simulink model "clv3d"  (Simulink 8.4)
settings: Solver=ode45  SolverMode=SingleTasking  StartTime=0.0  StopTime=30  RelTol=1e-3  AbsTol=1e-6
settings Model: Creator=The MathWorks Inc.  LastModifiedBy=gcampa  ExtModeTrigMode=oneshot  ExtModeArmWhenConnect=off
settings DataIOCC: ExternalInput=[]  InitialState=[]  LimitDataPoints=off  SaveOutput=off  SaveTime=off
settings OptimizationCC: BlockReduction=off  BooleanDataType=off  ExpressionDepthLimit=128  InitFltsAndDblsToZero=on
settings DebuggingCC: SaveWithParameterizedLinksMsg=none  SignalResolutionControl=TryResolveAllWithWarning  SolverPrmCheckMsg=none  MultiTaskDSMMsg=warning  MultiTaskCondExecSysMsg=none  IntegerOverflowMsg=none  FcnCallInpInsideContextMsg=EnableAllAsError  FrameProcessingCompatibilityMsg=error  StateNameClashWarn=none
settings HardwareCC: TargetUnknown=on
settings GRTTargetCC: TargetFcnLib=ansi_tfl_tmw.mat
settings ConfigComp: CovMetricSettings=dw  CovHtmlReporting=on  CovSaveCumulativeToWorkspaceVar=on  CovSaveSingleToWorkspaceVar=on  CovModelRefEnable=Off  CovExternalEMLEnable=off  CovSFcnEnable=off

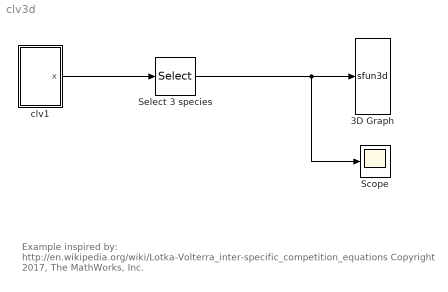
== system clv3d ==
  note: Example inspired by:
      | http://en.wikipedia.org/wiki/Lotka-Volterra_inter-specific_competition_equations
      | Copyright 2017, The MathWorks, Inc.
  3D Graph : S-Function  LoadFcn=if exist('sfun3d','file'), sfun3d([],[],[],'LoadBlock'); end  FunctionName=sfun3d  Parameters=ax,T,np,cp,gd,ls,mk,mx,hd,tb  EnableBusSupport=off  mask(3D Graph){np=1, ax=[0 1 0 1 0 0.5], mx=1e4, T=0.01, cp=[3 2 1], gd=on, hd=on, tb=on, ls=-, mk=none}
      mask prompts: np "Number of moving points (lines)"; ax "Range: [xmin xmax  ymin ymax zmin zmax]"; mx "Max number of points in each line"; T "Sampling Time"; cp "Camera position (use [0 0 1] for 2D XY view)"; gd "Grid (on|off)"; hd "HeadMarkers (on|off)"; tb "Toolbar (on|off)"; ls "LineStyle"; mk "LineMarker"
      mask help:
      | This block plots the position of several points in the XYZ space. The input contains the coordinates of all the points (x1,y1,z1,x2,y2,z2,...).
      | The number of moving points (lines), the XYZ ranges, sampling time, camera position, and grid (among other things) can be set as mask parameters.
      settings: CopyFcn=if exist('sfun3d','file'), sfun3d([],[],[],'CopyBlock'); end  DeleteFcn=if exist('sfun3d','file'), sfun3d([],[],[],'DeleteBlock'); end  NameChangeFcn=if exist('sfun3d','file'), sfun3d([],[],[],'NameChange'); end
      mask Help:
      | This block plots the position of several points in the XYZ space. The input contains the coordinates of all the points (x1,y1,z1,x2,y2,z2,...).
      | The number of moving points (lines), the XYZ ranges, sampling time, camera position, and grid (among other things) can be set as mask parameters.
      mask TypeOptions ls: - | -- | : | -. | none
      mask TypeOptions mk: none | . | + | o | * | x | square | diamond | v | ^ | > | < | pentagram | hexagram
      mask Display: plot([.05 .95 .95 .05 .05],[.45 .45 .95 .95 .45], 0.5+cos(0:0.1:2*pi)*0.3,0.7+sin(0:0.1:2*pi)*0.2)
  Scope : Scope
      settings: TimeRange=40  YMin=0  YMax=0.8
  Select 3 species : Selector  InputPortWidth=4  Indices=1:3
  clv1 : Subsystem  mask(Competitive Lotka Volterra System){A=[1 1.09 1.52 0; 0 1 0.44 1.36; 2.33 0 1 1.47; 1.21 0.51 0.35 1], R=diag([1 0.72 1.53 1.27]), x0=[0.2 0.2 0.2 0.1]}
      mask prompts: x0 "Initial Condition"
      mask help:
      | This autonomous system represents the competitive lotka volterra system
      |  xdot =  Rx .* ( 1 - Ax)
      |  where each component of x represents a population,
      |  A is an interaction matrix, and R is a diagonal "growth rate" matrix.
      |  Parameters and initial state can be selected from the mask.
      mask Help:
      | This autonomous system represents the competitive lotka volterra system
      |  <p>
      |  The system equations are:
      |  xdot =  Rx .* ( 1 - Ax)
      |  where each component of x represents a population,
      |  A is an interaction matrix, and R is a diagonal "growth rate" matrix.
      |  Parameters and initial state can be selected from the mask.
  wires:
  clv1/1(x) -> Select 3 species/1
  Select 3 species/1 -> 3D Graph/1, Scope/1

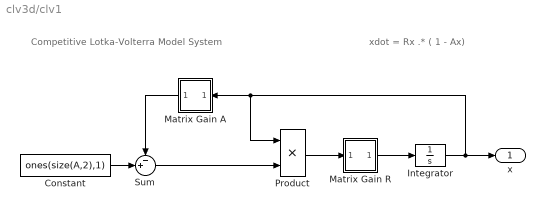
== system clv3d/clv1 ==
  note: Competitive Lotka-Volterra Model System
  note: xdot = Rx .* ( 1 - Ax)
  Constant : Constant  Value=ones(size(A,2),1)
  Integrator : Integrator  InitialCondition=x0
  Matrix Gain A : Subsystem  mask(Matrix Gain){K=A}
      mask prompts: K "Gain matrix:"
      mask help: Matrix Gain.
      mask Help: Multiplies input vector by entered matrix to produce output vector (y=Au).
      mask Display: disp('A')
  Matrix Gain R : Subsystem  mask(Matrix Gain){K=R}
      mask prompts: K "Gain matrix:"
      mask help: Matrix Gain.
      mask Help: Multiplies input vector by entered matrix to produce output vector (y=Au).
      mask Display: disp('R')
  Product : Product  SaturateOnIntegerOverflow=on  RndMeth=Zero  InputSameDT=on  OutDataTypeStr=Inherit: Same as first input
  Sum : Sum  Inputs=-+|  InputSameDT=on  OutDataTypeStr=Inherit: Same as first input
  x : Outport
  wires:
  Constant/1 -> Sum/2
  Matrix Gain A/1(Out1) -> Sum/1
  Sum/1 -> Product/2
  Integrator/1 -> x/1, Product/1, Matrix Gain A/1(In1)
  Product/1 -> Matrix Gain R/1(In1)
  Matrix Gain R/1(Out1) -> Integrator/1

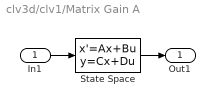
== system clv3d/clv1/Matrix Gain A ==
  In1 : Inport
  State Space : StateSpace  A=[]  B=[]  C=[]  D=K  X0=0
  Out1 : Outport
  wires:
  In1/1 -> State Space/1
  State Space/1 -> Out1/1

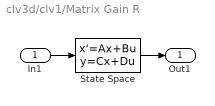
== system clv3d/clv1/Matrix Gain R ==
  In1 : Inport
  State Space : StateSpace  A=[]  B=[]  C=[]  D=K  X0=0
  Out1 : Outport
  wires:
  State Space/1 -> Out1/1
  In1/1 -> State Space/1
